simulink model "two_link_manipulator"  (R2021b)
settings: Solver=VariableStepAuto  StartTime=0.0  StopTime=20  RelTol=1e-3
settings Model: Creator=vkashyap  LastModifiedBy=vkashyap

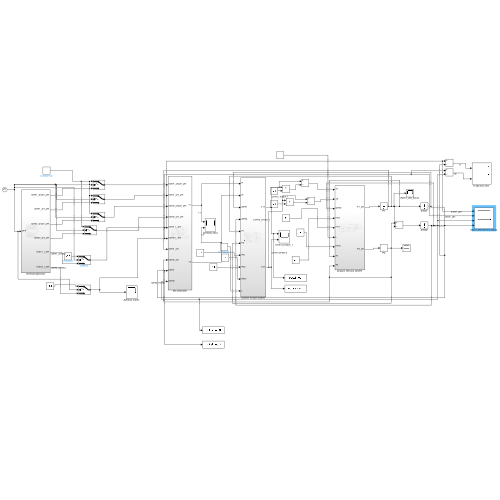
[thumbnail: Simulink's stored preview of the top-level diagram]
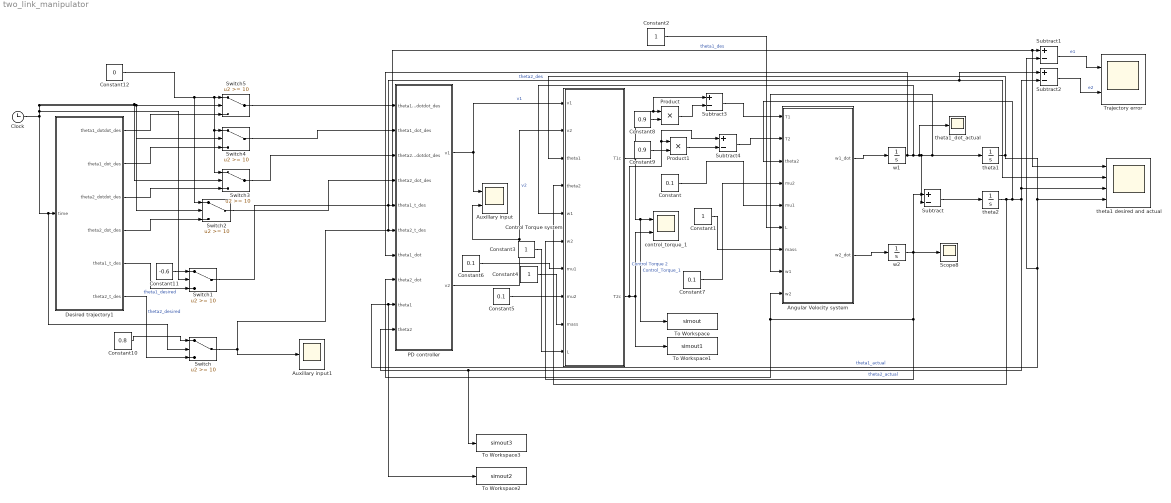
== system two_link_manipulator ==
  Angular Velocity system : Subsystem
  Auxillary input : Scope  NumInputPorts=2
  Auxillary input1 : Scope
  Clock : Clock
  Constant{,5..7} (4 alike) : Constant  Value=0.1
  Constant{1..4} (4 alike) : Constant
  Constant10 : Constant  Value=0.8
  Constant11 : Constant  Value=-0.6
  Constant12 : Constant  Value=0
  Constant8 : Constant  Value=0.9
  Constant9 : Constant  Value=0.9
  Control Torque system : Subsystem
  Desired trajectory1 : Subsystem
  PD controller : Subsystem
  Product : Product
  Product1 : Product
  Scope8 : Scope
  Subtract{,1..4} (5 alike) : Sum  Inputs=+-
  Switch{,1..5} (6 alike) : Switch  Threshold=10
  To Workspace : ToWorkspace  VariableName=simout  SampleTime=-1
  To Workspace1 : ToWorkspace  VariableName=simout1  SampleTime=-1
  To Workspace2 : ToWorkspace  VariableName=simout2  SampleTime=-1
  To Workspace3 : ToWorkspace  VariableName=simout3  SampleTime=-1
  Trajectory error : Scope  NumInputPorts=2
  control_torque_1 : Scope  NumInputPorts=2
  theta1 : Integrator  InitialCondition=1.0
  theta1 desired and actual : Scope  NumInputPorts=4
  theta1_dot_actual : Scope
  theta2 : Integrator
  w1 : Integrator
  w2 : Integrator
  wires:
  w1/1 -> PD controller/7(theta1_dot), Control Torque system/5(w1), theta1_dot_actual/1, theta1/1, Angular Velocity system/8(w1), Subtract/2
  w2/1 -> Control Torque system/6(w2), PD controller/8(theta2_dot), Angular Velocity system/9(w2), Scope8/1, Subtract/1
  Subtract/1 -> theta2/1
  Angular Velocity system/1(w1_dot) -> w1/1
  Angular Velocity system/2(w2_dot) -> w2/1
  theta2/1 -> Control Torque system/4(theta2), theta1 desired and actual/3, Subtract2/2, PD controller/10(theta2), To Workspace3/1, Angular Velocity system/3(theta2)  "theta2_actual"
  theta1/1 -> Subtract1/2, To Workspace2/1, PD controller/9(theta1), theta1 desired and actual/4, Control Torque system/3(theta1)  "theta1_actual"
  Control Torque system/1(T1c) -> Subtract3/1, Product/1, control_torque_1/1, To Workspace/1  "Control_Torque_1"
  Control Torque system/2(T2c) -> Subtract4/1, Product1/1, To Workspace1/1, control_torque_1/2  "Control Torque 2"
  PD controller/1(v1) -> Auxillary input/1, Control Torque system/1(v1)  "v1"
  PD controller/2(v2) -> Control Torque system/2(v2), Auxillary input/2  "v2"
  Constant/1 -> Angular Velocity system/5(mu1)
  Constant3/1 -> Control Torque system/10(L)
  Constant4/1 -> Control Torque system/9(mass)
  Constant7/1 -> Angular Velocity system/4(mu2)
  Constant5/1 -> Control Torque system/8(mu2)
  Constant6/1 -> Control Torque system/7(mu1)
  Subtract1/1 -> Trajectory error/1  "e1"
  Constant1/1 -> Angular Velocity system/7(mass)
  Subtract2/1 -> Trajectory error/2  "e2"
  Constant2/1 -> Angular Velocity system/6(L)
  Constant8/1 -> Product/2
  Constant9/1 -> Product1/2
  Product/1 -> Subtract3/2
  Subtract3/1 -> Angular Velocity system/1(T1)
  Product1/1 -> Subtract4/2
  Subtract4/1 -> Angular Velocity system/2(T2)
  Clock/1 -> Switch2/2, Switch3/2, Switch4/2, Switch5/2, Switch1/2, Switch/2, Desired trajectory1/1(time)
  Switch/1 -> Auxillary input1/1, Subtract2/1, theta1 desired and actual/2, PD controller/6(theta2_t_des)  "theta2_des"
  Desired trajectory1/6(theta2_t_des) -> Switch/3  "theta2_desired"
  Constant10/1 -> Switch/1
  Desired trajectory1/5(theta1_t_des) -> Switch1/3  "theta1_desired"
  Switch1/1 -> theta1 desired and actual/1, Subtract1/1, PD controller/5(theta1_t_des)  "theta1_des"
  Constant11/1 -> Switch1/1
  Desired trajectory1/1(theta1_dotdot_des) -> Switch5/3
  Switch5/1 -> PD controller/1(theta1_dotdot_des)
  Switch4/1 -> PD controller/2(theta1_dot_des)
  Desired trajectory1/2(theta1_dot_des) -> Switch4/3
  Switch3/1 -> PD controller/3(theta2_dotdot_des)
  Desired trajectory1/3(theta2_dotdot_des) -> Switch3/3
  Switch2/1 -> PD controller/4(theta2_dot_des)
  Desired trajectory1/4(theta2_dot_des) -> Switch2/3
  Constant12/1 -> Switch2/1, Switch4/1, Switch3/1, Switch5/1

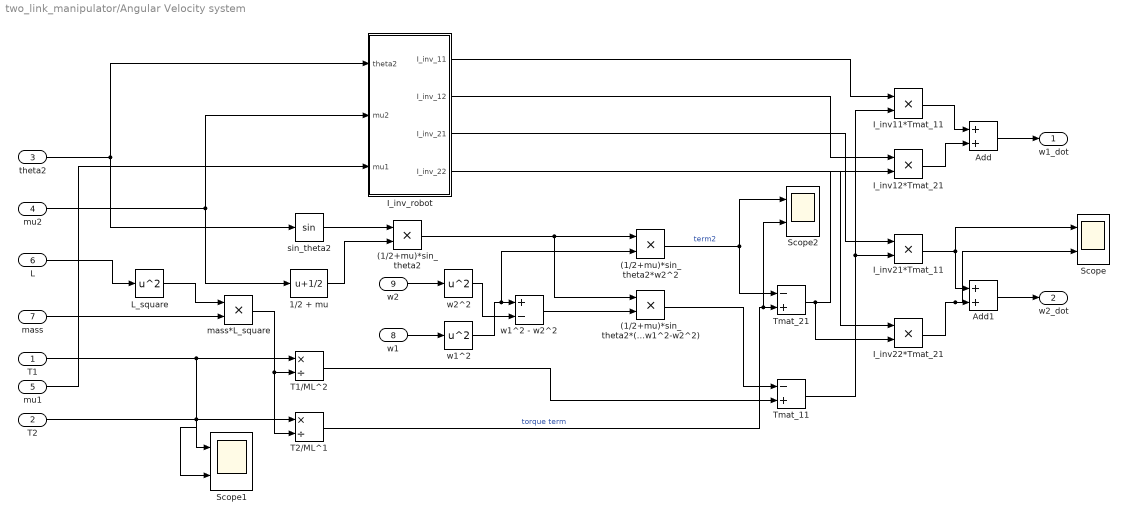
== system two_link_manipulator/Angular Velocity system ==
  T1 : Inport
  T2 : Inport  Port=2
  theta2 : Inport  Port=3
  mu2 : Inport  Port=4
  mu1 : Inport  Port=5
  L : Inport  Port=6
  mass : Inport  Port=7
  w1 : Inport  Port=8
  w2 : Inport  Port=9
  (1/2+mu)*sin_theta2 : Product
  (1/2+mu)*sin_theta2*(w1^2-w2^2) : Product
  (1/2+mu)*sin_theta2*w2^2 : Product
  1/2 + mu : Bias  Bias=1/2
  Add : Sum
  Add1 : Sum
  I_inv11*Tmat_11 : Product
  I_inv12*Tmat_21 : Product
  I_inv21*Tmat_11 : Product
  I_inv22*Tmat_21 : Product
  I_inv_robot : Subsystem
  L_square : Math  Operator=square  SaturateOnIntegerOverflow=on
  Scope : Scope  NumInputPorts=2
  Scope1 : Scope  NumInputPorts=2
  Scope2 : Scope  NumInputPorts=2
  T1/ML^2 : Product  Inputs=*/
  T2/ML^1 : Product  Inputs=*/
  Tmat_11 : Sum  Inputs=-+
  Tmat_21 : Sum  Inputs=-+
  mass*L_square : Product
  sin_theta2 : Trigonometry
  w1^2 : Math  Operator=square  SaturateOnIntegerOverflow=on
  w1^2 - w2^2 : Sum  Inputs=+-
  w2^2 : Math  Operator=square  SaturateOnIntegerOverflow=on
  w1_dot : Outport
  w2_dot : Outport  Port=2
  wires:
  theta2/1 -> sin_theta2/1, I_inv_robot/1(theta2)
  mu2/1 -> 1/2 + mu/1, I_inv_robot/2(mu2)
  L/1 -> L_square/1
  T1/1 -> Scope1/1, T1/ML^2/1
  mass*L_square/1 -> T2/ML^1/2, T1/ML^2/2
  T2/1 -> Scope1/2, T2/ML^1/1
  L_square/1 -> mass*L_square/1
  mass/1 -> mass*L_square/2
  sin_theta2/1 -> (1/2+mu)*sin_theta2/1
  1/2 + mu/1 -> (1/2+mu)*sin_theta2/2
  w2/1 -> w2^2/1
  w1/1 -> w1^2/1
  (1/2+mu)*sin_theta2/1 -> (1/2+mu)*sin_theta2*(w1^2-w2^2)/1, (1/2+mu)*sin_theta2*w2^2/1
  w2^2/1 -> w1^2 - w2^2/2
  w1^2/1 -> (1/2+mu)*sin_theta2*w2^2/2, w1^2 - w2^2/1
  w1^2 - w2^2/1 -> (1/2+mu)*sin_theta2*(w1^2-w2^2)/2
  T1/ML^2/1 -> Tmat_11/2
  (1/2+mu)*sin_theta2*(w1^2-w2^2)/1 -> Tmat_11/1
  (1/2+mu)*sin_theta2*w2^2/1 -> Scope2/1, Tmat_21/1  "term2"
  T2/ML^1/1 -> Scope2/2, Tmat_21/2  "torque term"
  I_inv_robot/1(I_inv_11) -> I_inv11*Tmat_11/1
  Tmat_11/1 -> I_inv21*Tmat_11/2, I_inv11*Tmat_11/2
  I_inv_robot/2(I_inv_12) -> I_inv12*Tmat_21/1
  Tmat_21/1 -> I_inv22*Tmat_21/2, I_inv12*Tmat_21/2
  I_inv_robot/3(I_inv_21) -> I_inv21*Tmat_11/1
  I_inv_robot/4(I_inv_22) -> I_inv22*Tmat_21/1
  I_inv11*Tmat_11/1 -> Add/1
  I_inv12*Tmat_21/1 -> Add/2
  I_inv21*Tmat_11/1 -> Add1/1, Scope/1
  I_inv22*Tmat_21/1 -> Scope/2, Add1/2
  Add/1 -> w1_dot/1
  Add1/1 -> w2_dot/1
  mu1/1 -> I_inv_robot/3(mu1)

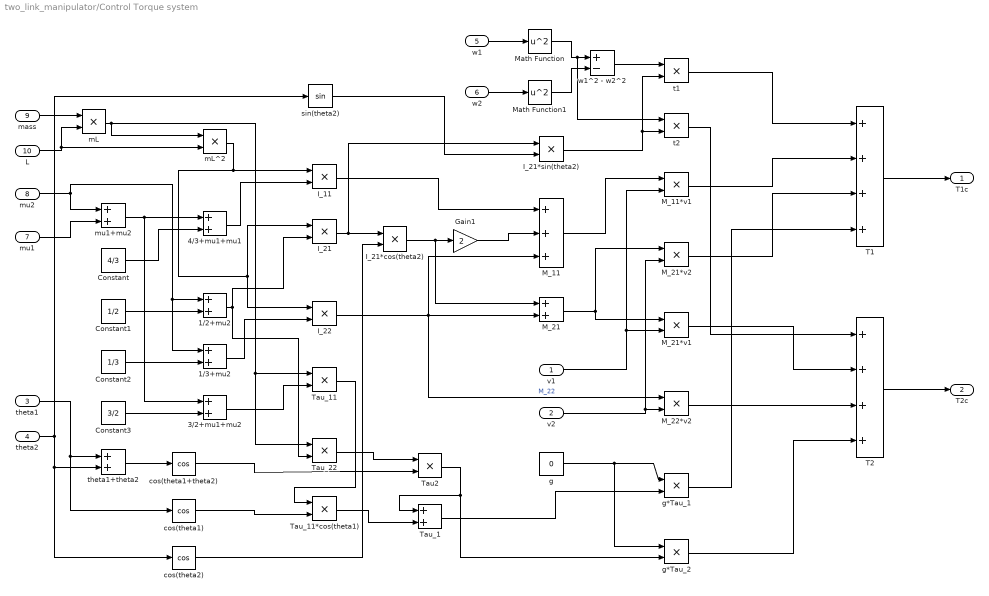
== system two_link_manipulator/Control Torque system ==
  v1 : Inport
  v2 : Inport  Port=2
  theta1 : Inport  Port=3
  theta2 : Inport  Port=4
  w1 : Inport  Port=5
  w2 : Inport  Port=6
  mu1 : Inport  Port=7
  mu2 : Inport  Port=8
  mass : Inport  Port=9
  L : Inport  Port=10
  1/2+mu2 : Sum
  1/3+mu2 : Sum
  3/2+mu1+mu2 : Sum
  4/3+mu1+mu1 : Sum
  Constant : Constant  Value=4/3
  Constant1 : Constant  Value=1/2
  Constant2 : Constant  Value=1/3
  Constant3 : Constant  Value=3/2
  Gain1 : Gain  Gain=2
  I_11 : Product
  I_21 : Product
  I_21*cos(theta2) : Product
  I_21*sin(theta2) : Product
  I_22 : Product
  M_11 : Sum  Inputs=+++
  M_11*v1 : Product
  M_21 : Sum
  M_21*v1 : Product
  M_21*v2 : Product
  M_22*v2 : Product
  Math Function : Math  Operator=square  SaturateOnIntegerOverflow=on
  Math Function1 : Math  Operator=square  SaturateOnIntegerOverflow=on
  T1 : Sum  Inputs=++++
  T2 : Sum  Inputs=++++
  Tau2 : Product
  Tau_1 : Sum
  Tau_11 : Product
  Tau_11*cos(theta1) : Product
  Tau_22 : Product
  cos(theta1) : Trigonometry  Operator=cos
  cos(theta1+theta2) : Trigonometry  Operator=cos
  cos(theta2) : Trigonometry  Operator=cos
  g : Constant  Value=0
  g*Tau_1 : Product
  g*Tau_2 : Product
  mL : Product
  mL^2 : Product
  mu1+mu2 : Sum
  sin(theta2) : Trigonometry
  t1 : Product
  t2 : Product
  theta1+theta2 : Sum
  w1^2 - w2^2 : Sum  Inputs=+-
  T1c : Outport
  T2c : Outport  Port=2
  wires:
  mass/1 -> mL/1
  L/1 -> mL^2/2, mL/2
  mL/1 -> Tau_22/1, Tau_11/1, mL^2/1
  mu2/1 -> mu1+mu2/1, 1/3+mu2/1, 1/2+mu2/1
  mu1/1 -> mu1+mu2/2
  mu1+mu2/1 -> 3/2+mu1+mu2/1, 4/3+mu1+mu1/1
  Constant/1 -> 4/3+mu1+mu1/2
  mL^2/1 -> I_22/1, I_21/1, I_11/1
  4/3+mu1+mu1/1 -> I_11/2
  Constant1/1 -> 1/2+mu2/2
  1/2+mu2/1 -> Tau_22/2, I_21/2
  Constant2/1 -> 1/3+mu2/2
  1/3+mu2/1 -> I_22/2
  Constant3/1 -> 3/2+mu1+mu2/2
  3/2+mu1+mu2/1 -> Tau_11/2
  Tau_22/1 -> Tau2/1
  theta1/1 -> cos(theta1)/1, theta1+theta2/1
  theta2/1 -> sin(theta2)/1, cos(theta2)/1, theta1+theta2/2
  theta1+theta2/1 -> cos(theta1+theta2)/1
  cos(theta1+theta2)/1 -> Tau2/2
  Tau_11/1 -> Tau_11*cos(theta1)/1
  cos(theta1)/1 -> Tau_11*cos(theta1)/2
  Tau2/1 -> g*Tau_2/2, Tau_1/1
  Tau_11*cos(theta1)/1 -> Tau_1/2
  I_21/1 -> I_21*sin(theta2)/1, I_21*cos(theta2)/1
  cos(theta2)/1 -> I_21*cos(theta2)/2
  I_22/1 -> M_22*v2/1, M_11/3, M_21/2  "M_22"
  I_21*cos(theta2)/1 -> Gain1/1, M_21/1
  Gain1/1 -> M_11/2
  I_11/1 -> M_11/1
  M_11/1 -> M_11*v1/1
  v1/1 -> M_21*v1/2, M_11*v1/2
  M_21/1 -> M_21*v1/1, M_21*v2/1
  v2/1 -> M_22*v2/2, M_21*v2/2
  sin(theta2)/1 -> I_21*sin(theta2)/2
  w1/1 -> Math Function/1
  w2/1 -> Math Function1/1
  Math Function/1 -> t2/1, w1^2 - w2^2/1
  Math Function1/1 -> w1^2 - w2^2/2
  w1^2 - w2^2/1 -> t1/1
  I_21*sin(theta2)/1 -> t2/2, t1/2
  g/1 -> g*Tau_2/1, g*Tau_1/1
  Tau_1/1 -> g*Tau_1/2
  t1/1 -> T1/1
  M_11*v1/1 -> T1/2
  M_21*v2/1 -> T1/3
  g*Tau_1/1 -> T1/4
  t2/1 -> T2/1
  M_21*v1/1 -> T2/2
  M_22*v2/1 -> T2/3
  g*Tau_2/1 -> T2/4
  T1/1 -> T1c/1
  T2/1 -> T2c/1

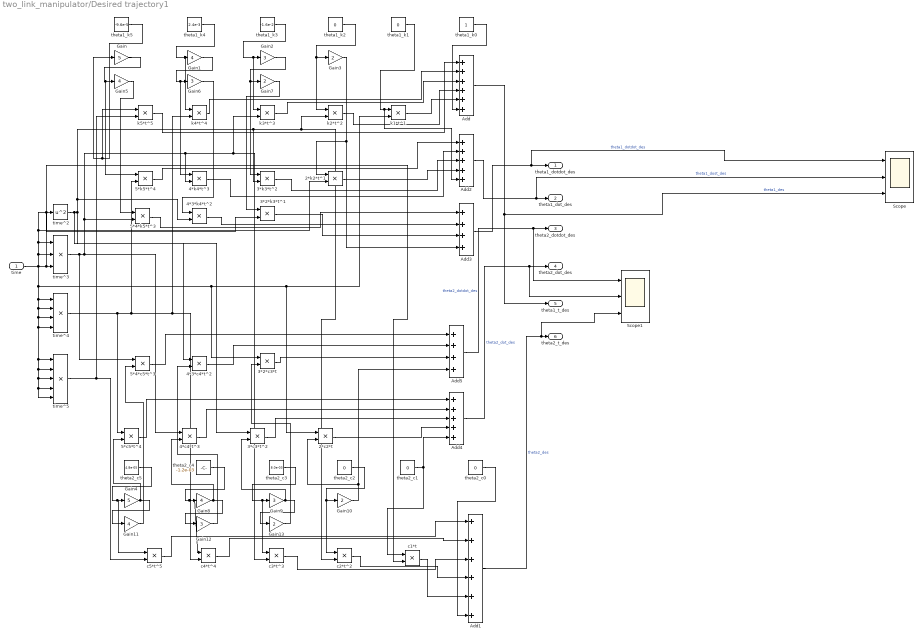
== system two_link_manipulator/Desired trajectory1 ==
  time : Inport
  2*c2*t : Product
  2*k2*t^1 : Product
  3*2*c3*t : Product
  3*2*k3*t^1 : Product
  3*c3*t^2 : Product
  3*k3*t^2 : Product
  4*3*c4*t^2 : Product
  4*3*k4*t^2 : Product
  4*c4*t^3 : Product
  4*k4*t^3 : Product
  5*4*c5*t^3 : Product
  5*4*k5*t^3 : Product
  5*c5*t^4 : Product
  5*k5*t^4 : Product
  Add : Sum  Inputs=++++++
  Add1 : Sum  Inputs=++++++
  Add2 : Sum  Inputs=+++++
  Add3 : Sum  Inputs=++++
  Add4 : Sum  Inputs=+++++
  Add5 : Sum  Inputs=++++
  Gain : Gain  Gain=5
  Gain{1,5,8,11} (4 alike) : Gain  Gain=4
  Gain{3,7,10,13} (4 alike) : Gain  Gain=2
  Gain{2,6,9,12} (4 alike) : Gain  Gain=3
  Gain4 : Gain  Gain=5
  Scope : Scope  NumInputPorts=3
  Scope1 : Scope  NumInputPorts=3
  c1*t : Product
  c2*t^2 : Product
  c3*t^3 : Product
  c4*t^4 : Product
  c5*t^5 : Product
  k1*t^1 : Product
  k2*t^2 : Product
  k3*t^3 : Product
  k4*t^4 : Product
  k5*t^5 : Product
  theta1_k0 : Constant
  theta1_k1 : Constant  Value=0
  theta1_k2 : Constant  Value=0
  theta1_k3 : Constant  Value=-1.6e-2
  theta1_k4 : Constant  Value=2.4e-3
  theta1_k5 : Constant  Value=-9.6e-5
  theta2_c0 : Constant  Value=0
  theta2_c1 : Constant  Value=0
  theta2_c2 : Constant  Value=0
  theta2_c3 : Constant  Value=8.0e-03
  theta2_c4 : Constant  Value=-1.2e-03
  theta2_c5 : Constant  Value=4.8e-05
  time^2 : Math  Operator=square  SaturateOnIntegerOverflow=on
  time^3 : Product  Inputs=3
  time^4 : Product  Inputs=4
  time^5 : Product  Inputs=5
  theta1_dotdot_des : Outport
  theta1_dot_des : Outport  Port=2
  theta2_dotdot_des : Outport  Port=3
  theta2_dot_des : Outport  Port=4
  theta1_t_des : Outport  Port=5
  theta2_t_des : Outport  Port=6
  wires:
  theta1_k5/1 -> Gain/1, k5*t^5/1
  theta1_k4/1 -> k4*t^4/1, Gain1/1
  theta1_k3/1 -> k3*t^3/1, Gain2/1
  theta1_k2/1 -> k2*t^2/1, Gain3/1
  theta1_k1/1 -> Add2/5, k1*t^1/1
  Gain/1 -> Gain5/1, 5*k5*t^4/1
  Gain1/1 -> 4*k4*t^3/1, Gain6/1
  Gain2/1 -> 3*k3*t^2/1, Gain7/1
  time/1 -> 3*2*c3*t/1, 2*c2*t/1, k1*t^1/2, time^4/4, time^5/1, time^5/2, time^5/3, time^5/4, time^5/5, time^4/3, time^4/2, time^4/1, c1*t/2, time^3/3, 2*k2*t^1/2, 3*2*k3*t^1/2, time^2/1, time^3/1, time^3/2
  time^5/1 -> c5*t^5/2, k5*t^5/2
  time^4/1 -> 5*c5*t^4/1, 5*k5*t^4/2, c4*t^4/2, k4*t^4/2
  time^3/1 -> 5*4*c5*t^3/1, 4*c4*t^3/1, 5*4*k5*t^3/2, 4*k4*t^3/2, c3*t^3/2, k3*t^3/2
  time^2/1 -> 4*3*c4*t^2/1, 3*c3*t^2/1, 4*3*k4*t^2/2, 3*k3*t^2/2, c2*t^2/2, k2*t^2/2
  k5*t^5/1 -> Add/1
  k4*t^4/1 -> Add/2
  k3*t^3/1 -> Add/3
  k2*t^2/1 -> Add/4
  k1*t^1/1 -> Add/5
  theta1_k0/1 -> Add/6
  Add/1 -> Scope/3, theta1_t_des/1  "theta1_des"
  theta2_c3/1 -> c3*t^3/1, Gain9/1
  theta2_c4/1 -> c4*t^4/1, Gain8/1
  theta2_c0/1 -> Add1/6
  theta2_c5/1 -> c5*t^5/1, Gain4/1
  theta2_c1/1 -> Add4/5, c1*t/1
  c4*t^4/1 -> Add1/2
  theta2_c2/1 -> c2*t^2/1, Gain10/1
  c3*t^3/1 -> Add1/3
  Gain8/1 -> 4*c4*t^3/2, Gain12/1
  c2*t^2/1 -> Add1/4
  Gain9/1 -> 3*c3*t^2/2, Gain13/1
  Gain4/1 -> 5*c5*t^4/2, Gain11/1
  c1*t/1 -> Add1/5
  c5*t^5/1 -> Add1/1
  Add1/1 -> Scope1/3, theta2_t_des/1  "theta2_des"
  Gain3/1 -> Add3/4, 2*k2*t^1/1
  5*k5*t^4/1 -> Add2/1
  4*k4*t^3/1 -> Add2/2
  3*k3*t^2/1 -> Add2/3
  2*k2*t^1/1 -> Add2/4
  Add2/1 -> Scope/2, theta1_dot_des/1  "theta1_dost_des"
  Gain5/1 -> 5*4*k5*t^3/1
  Gain6/1 -> 4*3*k4*t^2/1
  Gain7/1 -> 3*2*k3*t^1/1
  5*4*k5*t^3/1 -> Add3/1
  4*3*k4*t^2/1 -> Add3/2
  3*2*k3*t^1/1 -> Add3/3
  Add3/1 -> Scope/1, theta1_dotdot_des/1  "theta1_dotdot_des"
  Gain10/1 -> Add5/4, 2*c2*t/2
  5*c5*t^4/1 -> Add4/1
  4*c4*t^3/1 -> Add4/2
  3*c3*t^2/1 -> Add4/3
  2*c2*t/1 -> Add4/4
  Add4/1 -> theta2_dot_des/1, Scope1/2  "theta2_dot_des"
  Gain11/1 -> 5*4*c5*t^3/2
  Gain12/1 -> 4*3*c4*t^2/2
  Gain13/1 -> 3*2*c3*t/2
  5*4*c5*t^3/1 -> Add5/1
  4*3*c4*t^2/1 -> Add5/2
  3*2*c3*t/1 -> Add5/3
  Add5/1 -> theta2_dotdot_des/1, Scope1/1  "theta2_dotdot_des"

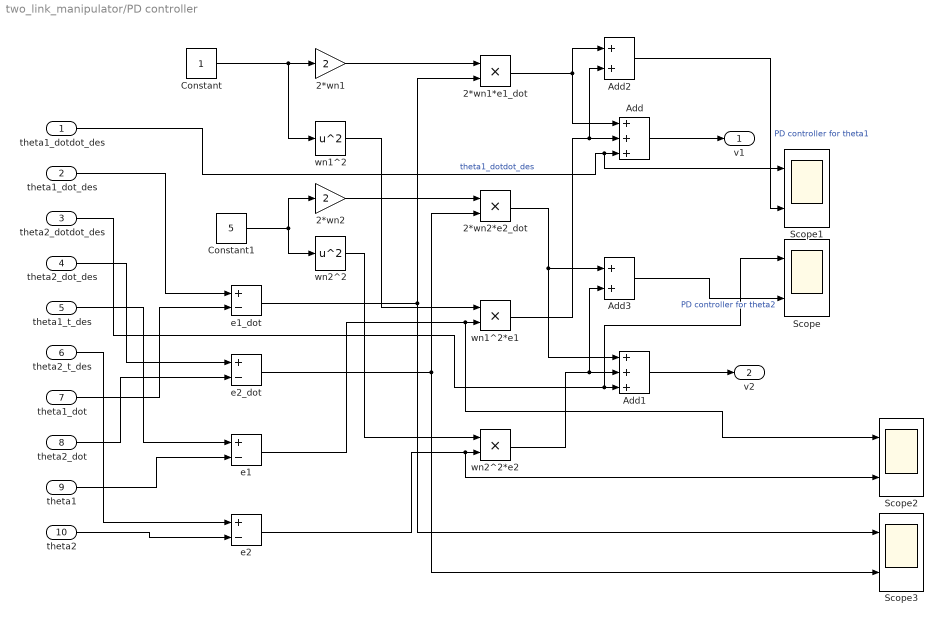
== system two_link_manipulator/PD controller ==
  theta1_dotdot_des : Inport
  theta1_dot_des : Inport  Port=2
  theta2_dotdot_des : Inport  Port=3
  theta2_dot_des : Inport  Port=4
  theta1_t_des : Inport  Port=5
  theta2_t_des : Inport  Port=6
  theta1_dot : Inport  Port=7
  theta2_dot : Inport  Port=8
  theta1 : Inport  Port=9
  theta2 : Inport  Port=10
  2*wn1 : Gain  Gain=2
  2*wn1*e1_dot : Product
  2*wn2 : Gain  Gain=2
  2*wn2*e2_dot : Product
  Add : Sum  Inputs=+++
  Add1 : Sum  Inputs=+++
  Add2 : Sum
  Add3 : Sum
  Constant : Constant  VectorParams1D=off
  Constant1 : Constant  Value=5  VectorParams1D=off
  Scope{,1..3} (4 alike) : Scope  NumInputPorts=2
  e1 : Sum  Inputs=+-
  e1_dot : Sum  Inputs=+-
  e2 : Sum  Inputs=+-
  e2_dot : Sum  Inputs=+-
  wn1^2 : Math  Operator=square  SaturateOnIntegerOverflow=on
  wn1^2*e1 : Product
  wn2^2 : Math  Operator=square  SaturateOnIntegerOverflow=on
  wn2^2*e2 : Product
  v1 : Outport
  v2 : Outport  Port=2
  wires:
  Constant1/1 -> 2*wn2/1, wn2^2/1
  Constant/1 -> wn1^2/1, 2*wn1/1
  theta1_dot_des/1 -> e1_dot/1
  theta1_dot/1 -> e1_dot/2
  theta2_dot_des/1 -> e2_dot/1
  theta2_dot/1 -> e2_dot/2
  theta1_t_des/1 -> e1/1
  theta1/1 -> e1/2
  theta2/1 -> e2/2
  theta2_t_des/1 -> e2/1
  2*wn1/1 -> 2*wn1*e1_dot/1
  e1_dot/1 -> Scope3/1, 2*wn1*e1_dot/2
  2*wn2/1 -> 2*wn2*e2_dot/1
  e2_dot/1 -> Scope3/2, 2*wn2*e2_dot/2
  wn1^2/1 -> wn1^2*e1/1
  e1/1 -> Scope2/1, wn1^2*e1/2
  wn2^2/1 -> wn2^2*e2/1
  e2/1 -> Scope2/2, wn2^2*e2/2
  2*wn1*e1_dot/1 -> Add2/1, Add/1
  wn1^2*e1/1 -> Add2/2, Add/2
  theta1_dotdot_des/1 -> Scope1/1, Add/3  "theta1_dotdot_des"
  2*wn2*e2_dot/1 -> Add3/1, Add1/1
  wn2^2*e2/1 -> Add3/2, Add1/2
  theta2_dotdot_des/1 -> Scope/1, Add1/3
  Add/1 -> v1/1
  Add1/1 -> v2/1
  Add2/1 -> Scope1/2  "PD controller for theta1"
  Add3/1 -> Scope/2  "PD controller for theta2"

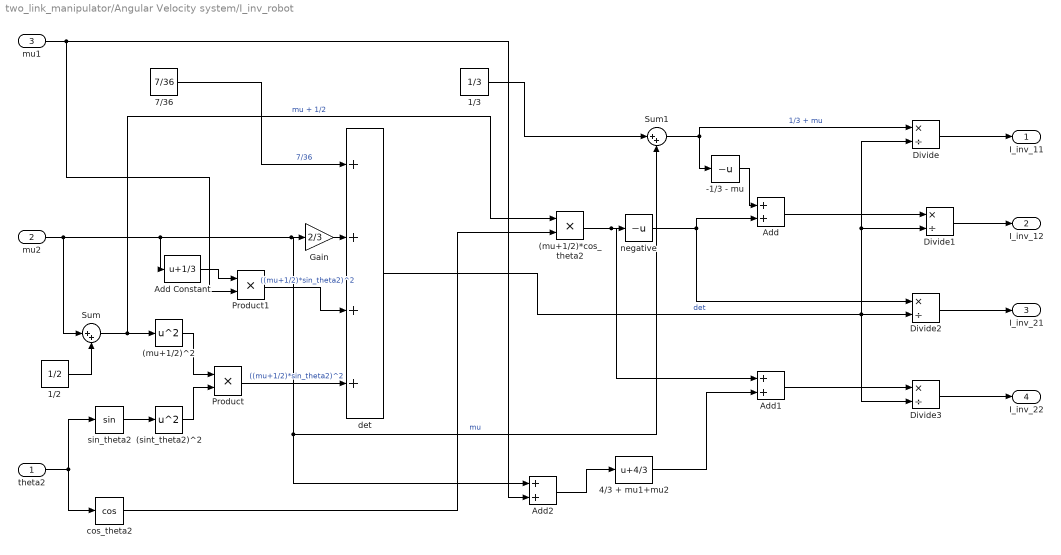
== system two_link_manipulator/Angular Velocity system/I_inv_robot ==
  theta2 : Inport
  mu2 : Inport  Port=2
  mu1 : Inport  Port=3
  (mu+1/2)*cos_theta2 : Product
  (mu+1/2)^2 : Math  Operator=square  SaturateOnIntegerOverflow=on
  (sint_theta2)^2 : Math  Operator=square  SaturateOnIntegerOverflow=on
  -1/3 - mu : UnaryMinus
  1/2 : Constant  Value=1/2
  1/3 : Constant  Value=1/3
  4/3 + mu1+mu2 : Bias  Bias=4/3
  7/36 : Constant  Value=7/36
  Add : Sum
  Add Constant : Bias  Bias=1/3
  Add1 : Sum
  Add2 : Sum
  Divide{,1..3} (4 alike) : Product  Inputs=*/
  Gain : Gain  Gain=2/3
  Product : Product
  Product1 : Product
  Sum : Sum  Inputs=|++
  Sum1 : Sum  Inputs=|++
  cos_theta2 : Trigonometry  Operator=cos
  det : Sum  Inputs=++++
  negative : UnaryMinus
  sin_theta2 : Trigonometry
  I_inv_11 : Outport
  I_inv_12 : Outport  Port=2
  I_inv_21 : Outport  Port=3
  I_inv_22 : Outport  Port=4
  wires:
  7/36/1 -> det/1  "7/36"
  mu2/1 -> Sum/1, Add Constant/1, Add2/1, Sum1/2, Gain/1  "mu"
  1/2/1 -> Sum/2
  Sum/1 -> (mu+1/2)*cos_theta2/1, (mu+1/2)^2/1  "mu + 1/2"
  theta2/1 -> cos_theta2/1, sin_theta2/1
  sin_theta2/1 -> (sint_theta2)^2/1
  (sint_theta2)^2/1 -> Product/2
  (mu+1/2)^2/1 -> Product/1
  Product/1 -> det/4  "((mu+1/2)*sin_theta2)^2"
  1/3/1 -> Sum1/1
  Sum1/1 -> Divide/1, -1/3 - mu/1  "1/3 + mu"
  cos_theta2/1 -> (mu+1/2)*cos_theta2/2
  (mu+1/2)*cos_theta2/1 -> Add1/1, negative/1
  -1/3 - mu/1 -> Add/1
  negative/1 -> Divide2/1, Add/2
  Add/1 -> Divide1/1
  Add1/1 -> Divide3/1
  4/3 + mu1+mu2/1 -> Add1/2
  det/1 -> Divide3/2, Divide/2, Divide1/2, Divide2/2  "det"
  Divide2/1 -> I_inv_21/1
  Divide1/1 -> I_inv_12/1
  Divide/1 -> I_inv_11/1
  Divide3/1 -> I_inv_22/1
  mu1/1 -> Product1/2, Add2/2
  Add2/1 -> 4/3 + mu1+mu2/1
  Gain/1 -> det/2
  Add Constant/1 -> Product1/1
  Product1/1 -> det/3  "((mu+1/2)*sin_theta2)^2"
